simulink model "openMHA_test_ar_filter_dualport"  (R2020a)
settings: Solver=VariableStepAuto  StartTime=0.0  StopTime=stop_time  RelTol=1e-3
InitFcn:
  | test_ar_filter_dualport_init
StopFcn:
  | test_ar_filter_dualport_stop
values from neighbouring files (symbols this model uses):
  buf_a = 65.*ones(num_bands,1)    [test_FFT_to_gain_init.m]    (also in test_ar_filter_dualport_init.m; test_db_ar_gaintable_init.m)
  num_bands = 8    [calculate_gaintable.m]    (also in test_FFT_to_gain_init.m = 2; test_ar_filter_dualport_init.m = 2; test_db_ar_gaintable_init.m = 2; test_db_lookup_gain_fpga_init.m = 9)
libraries: dspsrcs4 x7, FPGA_Open_Speech_Tools x1, simulink x1
settings Model: PacingRate=1000  Creator=t96f346  LastModifiedBy=t96f346

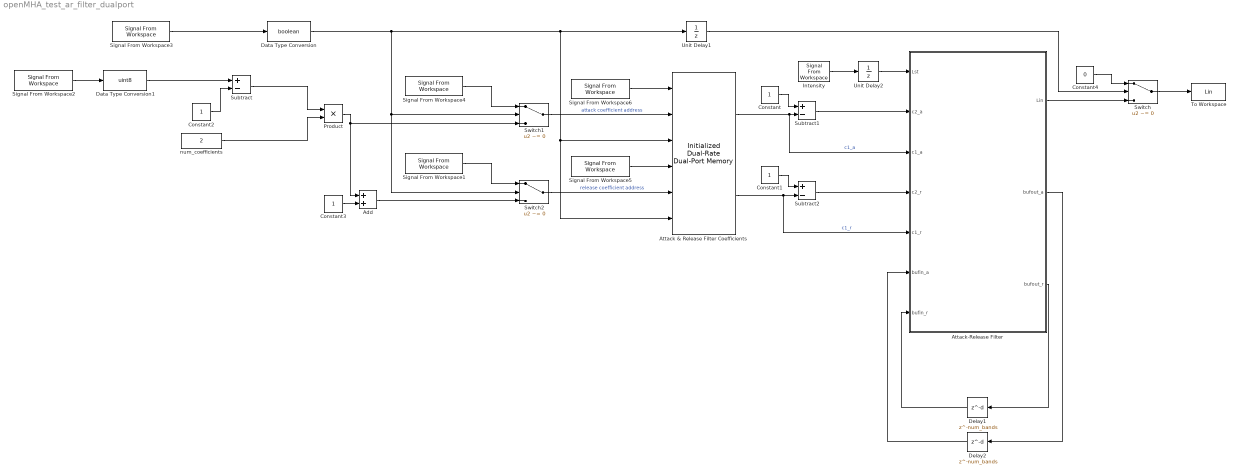
== system openMHA_test_ar_filter_dualport ==
  Add : Sum
  Attack & Release Filter Coefficients : FPGA_Open_Speech_Tools/Initialized Dual-Rate Dual-Port Memory  ram_size=coeff_size  Table_Init=ar_coeffs
      settings: SourceProductName=FPGA Open Speech Tools
  Attack-Release Filter : Subsystem
  Constant : Constant  SampleTime=-1
  Constant1 : Constant  SampleTime=-1
  Constant2 : Constant  OutDataTypeStr=uint8  SampleTime=-1
  Constant3 : Constant  SampleTime=-1
  Constant4 : Constant  Value=0  OutDataTypeStr=double  SampleTime=-1
  Data Type Conversion : DataTypeConversion  OutDataTypeStr=boolean
  Data Type Conversion1 : DataTypeConversion  OutDataTypeStr=uint8
  Delay1 : Delay  DelayLength=num_bands  InitialCondition=buf_a  UseCircularBuffer=on
  Delay2 : Delay  DelayLength=num_bands  InitialCondition=buf_a  UseCircularBuffer=on
  Intensity : dspsrcs4/Signal From Workspace  X=Lst  Ts=1  nsamps=1  OutputAfterFinalValue=Setting to zero  ignoreOrWarnInputAndFrameLengths=off  OutputFrames=off
  Product : Product  OutDataTypeStr=Inherit: Same as first input
  Signal From Workspace1 : dspsrcs4/Signal From Workspace  X=write_addrB  Ts=1  nsamps=1  OutputAfterFinalValue=Setting to zero  ignoreOrWarnInputAndFrameLengths=off  OutputFrames=off
  Signal From Workspace2 : dspsrcs4/Signal From Workspace  X=band_num  Ts=1  nsamps=1  OutputAfterFinalValue=Setting to zero  ignoreOrWarnInputAndFrameLengths=off  OutputFrames=off
  Signal From Workspace3 : dspsrcs4/Signal From Workspace  X=write_en  Ts=1  nsamps=1  OutputAfterFinalValue=Setting to zero  ignoreOrWarnInputAndFrameLengths=off  OutputFrames=off
  Signal From Workspace4 : dspsrcs4/Signal From Workspace  X=write_addrA  Ts=1  nsamps=1  OutputAfterFinalValue=Setting to zero  ignoreOrWarnInputAndFrameLengths=off  OutputFrames=off
  Signal From Workspace5 : dspsrcs4/Signal From Workspace  X=write_dataB  Ts=1  nsamps=1  OutputAfterFinalValue=Setting to zero  ignoreOrWarnInputAndFrameLengths=off  OutputFrames=off
  Signal From Workspace6 : dspsrcs4/Signal From Workspace  X=write_dataA  Ts=1  nsamps=1  OutputAfterFinalValue=Setting to zero  ignoreOrWarnInputAndFrameLengths=off  OutputFrames=off
  Subtract : Sum  Inputs=+-
  Subtract1 : Sum  Inputs=+-
  Subtract2 : Sum  Inputs=+-
  Switch : Switch  Criteria=u2 ~= 0  OutDataTypeStr=double
  Switch1 : Switch  Criteria=u2 ~= 0  OutDataTypeStr=uint8
  Switch2 : Switch  Criteria=u2 ~= 0  OutDataTypeStr=uint8
  To Workspace : ToWorkspace  VariableName=Lin  SampleTime=-1
      settings: Save2DSignal=2-D array (concatenate along first dimension)
  Unit Delay1 : UnitDelay  SampleTime=-1  HasFrameUpgradeWarning=on
  Unit Delay2 : UnitDelay  SampleTime=-1  HasFrameUpgradeWarning=on
  num_coefficients : Constant  Value=2  OutDataTypeStr=uint8  SampleTime=-1
  wires:
  Signal From Workspace2/1 -> Data Type Conversion1/1
  num_coefficients/1 -> Product/2
  Subtract/1 -> Product/1
  Constant2/1 -> Subtract/2
  Product/1 -> Switch1/3, Add/1
  Attack & Release Filter Coefficients/2 -> Attack-Release Filter/5(c1_r), Subtract2/2  "c1_r"
  Attack & Release Filter Coefficients/1 -> Attack-Release Filter/3(c1_a), Subtract1/2  "c1_a"
  Constant/1 -> Subtract1/1
  Constant1/1 -> Subtract2/1
  Subtract2/1 -> Attack-Release Filter/4(c2_r)
  Subtract1/1 -> Attack-Release Filter/2(c2_a)
  Add/1 -> Switch2/3
  Constant3/1 -> Add/2
  Signal From Workspace3/1 -> Data Type Conversion/1
  Data Type Conversion/1 -> Unit Delay1/1, Attack & Release Filter Coefficients/3, Attack & Release Filter Coefficients/6, Switch1/2, Switch2/2
  Switch/1 -> To Workspace/1
  Constant4/1 -> Switch/1
  Attack-Release Filter/1(Lin) -> Switch/3
  Switch2/1 -> Attack & Release Filter Coefficients/5  "release coefficient address"
  Switch1/1 -> Attack & Release Filter Coefficients/2  "attack coefficient address"
  Intensity/1 -> Unit Delay2/1
  Unit Delay1/1 -> Switch/2
  Signal From Workspace4/1 -> Switch1/1
  Signal From Workspace1/1 -> Switch2/1
  Data Type Conversion1/1 -> Subtract/1
  Signal From Workspace6/1 -> Attack & Release Filter Coefficients/1
  Signal From Workspace5/1 -> Attack & Release Filter Coefficients/4
  Attack-Release Filter/3(bufout_r) -> Delay1/1
  Delay1/1 -> Attack-Release Filter/7(bufin_r)
  Attack-Release Filter/2(bufout_a) -> Delay2/1
  Delay2/1 -> Attack-Release Filter/6(bufin_a)
  Unit Delay2/1 -> Attack-Release Filter/1(Lst)

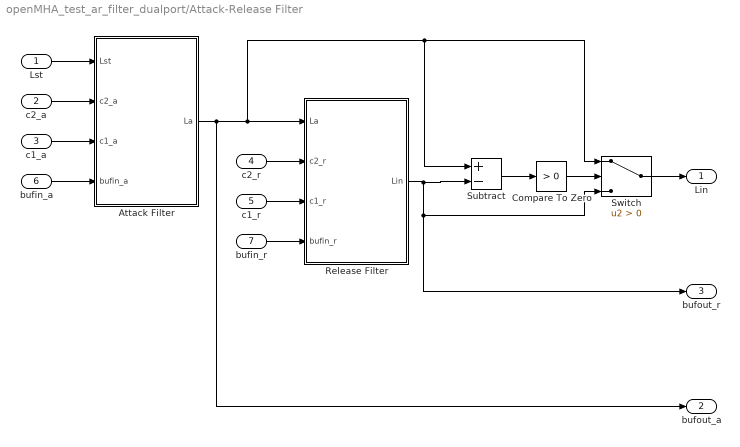
== system openMHA_test_ar_filter_dualport/Attack-Release Filter ==
  Lst : Inport
  c2_a : Inport  Port=2
  c1_a : Inport  Port=3
  c2_r : Inport  Port=4
  c1_r : Inport  Port=5
  bufin_a : Inport  Port=6
  bufin_r : Inport  Port=7
  Attack Filter : Subsystem  TreatAsAtomicUnit=on
  Compare To Zero : simulink/Logic and Bit Operations/Compare To Zero  relop=>  OutDataTypeStr=boolean
  Release Filter : Subsystem  TreatAsAtomicUnit=on
  Subtract : Sum  Inputs=+-  OutDataTypeStr=Inherit: Same as accumulator
  Switch : Switch  Criteria=u2 > Threshold
  Lin : Outport  VectorParamsAs1DForOutWhenUnconnected=off
  bufout_a : Outport  Port=2  VectorParamsAs1DForOutWhenUnconnected=off
  bufout_r : Outport  Port=3  VectorParamsAs1DForOutWhenUnconnected=off
  wires:
  Lst/1 -> Attack Filter/1(Lst)
  c2_a/1 -> Attack Filter/2(c2_a)
  c1_a/1 -> Attack Filter/3(c1_a)
  bufin_a/1 -> Attack Filter/4(bufin_a)
  c2_r/1 -> Release Filter/2(c2_r)
  c1_r/1 -> Release Filter/3(c1_r)
  bufin_r/1 -> Release Filter/4(bufin_r)
  Attack Filter/1(La) -> bufout_a/1, Switch/1, Subtract/1, Release Filter/1(La)
  Compare To Zero/1 -> Switch/2
  Release Filter/1(Lin) -> Subtract/2, Switch/3, bufout_r/1
  Subtract/1 -> Compare To Zero/1
  Switch/1 -> Lin/1

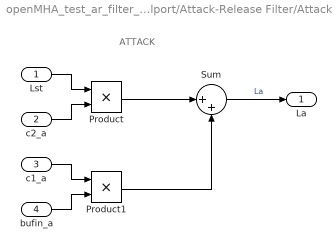
== system openMHA_test_ar_filter_dualport/Attack-Release Filter/Attack Filter ==
  note: ATTACK
  Lst : Inport
  c2_a : Inport  Port=2
  c1_a : Inport  Port=3
  bufin_a : Inport  Port=4
  Product : Product
  Product1 : Product
  Sum : Sum  Inputs=|++
  La : Outport  InitialOutput=0  VectorParamsAs1DForOutWhenUnconnected=off
  wires:
  Lst/1 -> Product/1
  Product/1 -> Sum/1
  Sum/1 -> La/1  "La"
  bufin_a/1 -> Product1/2
  Product1/1 -> Sum/2
  c2_a/1 -> Product/2
  c1_a/1 -> Product1/1

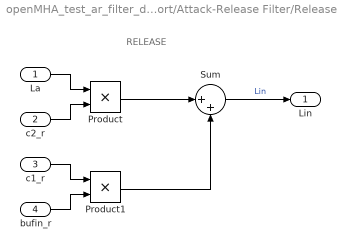
== system openMHA_test_ar_filter_dualport/Attack-Release Filter/Release Filter ==
  note: RELEASE
  La : Inport
  c2_r : Inport  Port=2
  c1_r : Inport  Port=3
  bufin_r : Inport  Port=4
  Product : Product
  Product1 : Product
  Sum : Sum  Inputs=|++
  Lin : Outport  InitialOutput=0  VectorParamsAs1DForOutWhenUnconnected=off
  wires:
  Sum/1 -> Lin/1  "Lin"
  c2_r/1 -> Product/2
  c1_r/1 -> Product1/1
  La/1 -> Product/1
  Product1/1 -> Sum/2
  Product/1 -> Sum/1
  bufin_r/1 -> Product1/2
